simulink model "MPC_states_constrained"  (R2024b)
settings: Solver=VariableStepAuto  StartTime=0.0  StopTime=tsim  RelTol=1e-3
values from neighbouring files (symbols this model uses):
  C_state = eye(12)    [main.m]
  D_state = zeros(12, 1)    [main.m]
  Q_LQ = q * eye(12)    [main.m]
  R_LQ = r    (= 1e-05)    [main.m]
  S = zeros(n)    [main.m]
  Ts = 0.1    [main.m]    (also in point7.m)
  Ubar_z = inv(dcgain(Gz))*Ybar    [main.m]
  umax = +15    (= 15)    [main.m]
  umin = -15    [main.m]
  x0 = [3,0,3,0,3,0,3,0,3,0,3,0]    [main.m]
  Xbar_z = (eye(12) - Az) \ (Bz * Ubar_z)    [main.m]
  xmax = [ 10;  Inf;  10;  Inf;  10;  Inf;  10;  Inf;  10;  Inf;  10;  Inf]    [main.m]
  xmin = [-10; -Inf; -10; -Inf; -10; -Inf; -10; -Inf; -10; -Inf; -10; -Inf]    [main.m]
undefined symbols (not defined in the file or in its folder): Az, Bz, Cz, mympc_project_constraints
settings Model: Creator=faiol  LastModifiedBy=faiol

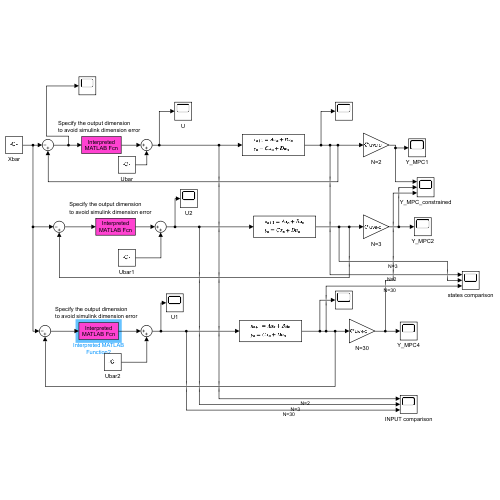
[thumbnail: Simulink's stored preview of the top-level diagram]
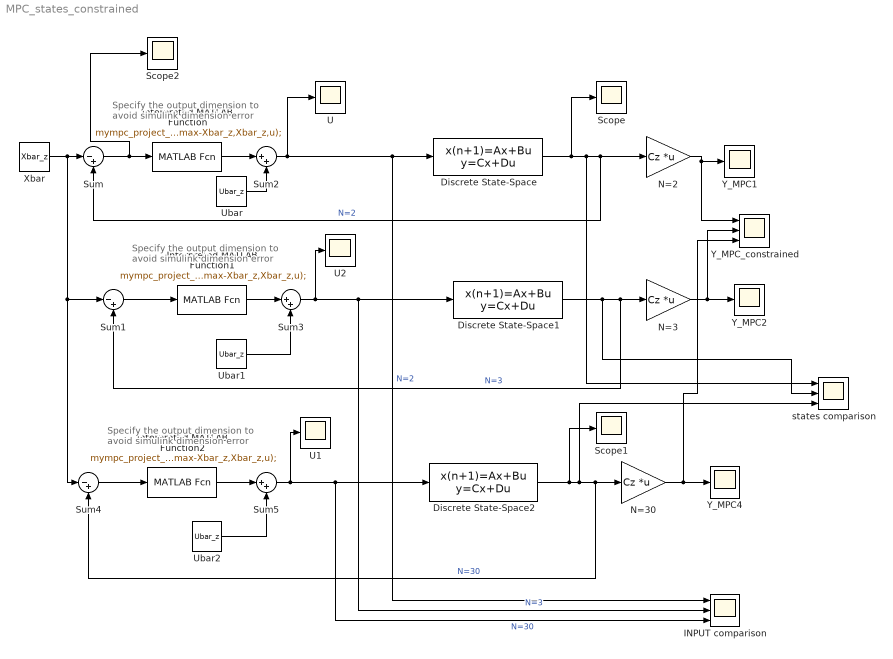
== system MPC_states_constrained ==
  note: Specify the output dimension
      | to avoid simulink dimension error
  note: Specify the output dimension
      | to avoid simulink dimension error
  note: Specify the output dimension
      | to avoid simulink dimension error
  Discrete State-Space : DiscreteStateSpace  A=Az  B=Bz  C=C_state  D=D_state  InitialCondition=x0  SampleTime=Ts
  Discrete State-Space1 : DiscreteStateSpace  A=Az  B=Bz  C=C_state  D=D_state  InitialCondition=x0  SampleTime=Ts
  Discrete State-Space2 : DiscreteStateSpace  A=Az  B=Bz  C=C_state  D=D_state  InitialCondition=x0  SampleTime=Ts
  INPUT comparison : Scope  NumInputPorts=3
  Interpreted MATLAB Function : MATLABFcn  MATLABFcn=mympc_project_constraints(Az,Bz,Q_LQ,R_LQ,S,2,umin-Ubar_z,umax-Ubar_z,Ubar_z,xmin-Xbar_z,xmax-Xbar_z,Xbar_z,u);  OutputDimensions=1
  Interpreted MATLAB Function1 : MATLABFcn  MATLABFcn=mympc_project_constraints(Az,Bz,Q_LQ,R_LQ,S,3,umin-Ubar_z,umax-Ubar_z,Ubar_z,xmin-Xbar_z,xmax-Xbar_z,Xbar_z,u);  OutputDimensions=1
  Interpreted MATLAB Function2 : MATLABFcn  MATLABFcn=mympc_project_constraints(Az,Bz,Q_LQ,R_LQ,S,30,umin-Ubar_z,umax-Ubar_z,Ubar_z,xmin-Xbar_z,xmax-Xbar_z,Xbar_z,u);  OutputDimensions=1
  N=2 : Gain  Gain=Cz  Multiplication=Matrix(K*u) (u vector)
  N=3 : Gain  Gain=Cz  Multiplication=Matrix(K*u) (u vector)
  N=30 : Gain  Gain=Cz  Multiplication=Matrix(K*u) (u vector)
  Scope : Scope
  Scope1 : Scope
  Scope2 : Scope
  Sum : Sum  Inputs=|-+
  Sum1 : Sum  Inputs=|-+
  Sum2 : Sum  Inputs=|++
  Sum3 : Sum  Inputs=|++
  Sum4 : Sum  Inputs=|-+
  Sum5 : Sum  Inputs=|++
  U : Scope
  U1 : Scope
  U2 : Scope
  Ubar : Constant  Value=Ubar_z  SampleTime=Ts
  Ubar1 : Constant  Value=Ubar_z  SampleTime=Ts
  Ubar2 : Constant  Value=Ubar_z  SampleTime=Ts
  Xbar : Constant  Value=Xbar_z  SampleTime=Ts
  Y_MPC1 : Scope
  Y_MPC2 : Scope
  Y_MPC4 : Scope
  Y_MPC_constrained : Scope  NumInputPorts=3
  states comparison : Scope  NumInputPorts=3
  wires:
  Discrete State-Space/1 -> Scope/1, states comparison/1, Sum/2, N=2/1  "N=2"
  Xbar/1 -> Sum4/1, Sum1/1, Sum/1
  N=3/1 -> Y_MPC_constrained/2, Y_MPC2/1
  Discrete State-Space1/1 -> states comparison/2, Sum1/2, N=3/1  "N=3"
  N=2/1 -> Y_MPC_constrained/1, Y_MPC1/1
  Sum/1 -> Scope2/1, Interpreted MATLAB Function/1
  Sum1/1 -> Interpreted MATLAB Function1/1
  Interpreted MATLAB Function/1 -> Sum2/1
  Ubar/1 -> Sum2/2
  Sum2/1 -> INPUT comparison/1, Discrete State-Space/1, U/1  "N=2"
  Sum3/1 -> INPUT comparison/2, Discrete State-Space1/1, U2/1  "N=3"
  Interpreted MATLAB Function1/1 -> Sum3/1
  Ubar1/1 -> Sum3/2
  Interpreted MATLAB Function2/1 -> Sum5/1
  Sum4/1 -> Interpreted MATLAB Function2/1
  Discrete State-Space2/1 -> Scope1/1, states comparison/3, Sum4/2, N=30/1  "N=30"
  N=30/1 -> Y_MPC_constrained/3, Y_MPC4/1
  Ubar2/1 -> Sum5/2
  Sum5/1 -> INPUT comparison/3, Discrete State-Space2/1, U1/1  "N=30"
